simulink model "SistemaSeguimientoConIntegrador"  (R2020a)
settings: Solver=VariableStepAuto  StartTime=0.0  StopTime=10  RelTol=1e-3
settings Model: Creator=Sergio  LastModifiedBy=Sergio

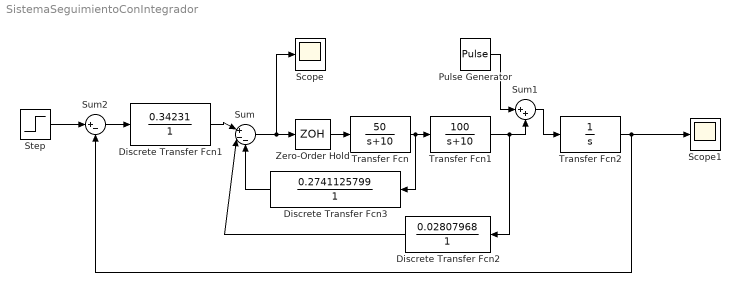
== system SistemaSeguimientoConIntegrador ==
  Discrete Transfer Fcn1 : DiscreteTransferFcn  Numerator=[0.34231]  Denominator=[1]
  Discrete Transfer Fcn2 : DiscreteTransferFcn  Numerator=[0.02807968]  Denominator=[1]
  Discrete Transfer Fcn3 : DiscreteTransferFcn  Numerator=[0.2741125799]  Denominator=[1]
  Pulse Generator : DiscretePulseGenerator  PulseType=Time based  Amplitude=0.1  Period=10
  Scope : Scope
  Scope1 : Scope
  Step : Step  SampleTime=0
  Sum : Sum  Inputs=|+--
  Sum1 : Sum  Inputs=|++
  Sum2 : Sum  Inputs=|+-
  Transfer Fcn : TransferFcn  Numerator=[50]  Denominator=[1 10]
  Transfer Fcn1 : TransferFcn  Numerator=[100]  Denominator=[1 10]
  Transfer Fcn2 : TransferFcn  Denominator=[1 0]
  Zero-Order Hold : ZeroOrderHold  SampleTime=0.02
  wires:
  Zero-Order Hold/1 -> Transfer Fcn/1
  Transfer Fcn/1 -> Discrete Transfer Fcn3/1, Transfer Fcn1/1
  Sum/1 -> Scope/1, Zero-Order Hold/1
  Transfer Fcn2/1 -> Sum2/2, Scope1/1
  Transfer Fcn1/1 -> Discrete Transfer Fcn2/1, Sum1/2
  Sum1/1 -> Transfer Fcn2/1
  Discrete Transfer Fcn3/1 -> Sum/3
  Discrete Transfer Fcn2/1 -> Sum/2
  Pulse Generator/1 -> Sum1/1
  Sum2/1 -> Discrete Transfer Fcn1/1
  Step/1 -> Sum2/1
  Discrete Transfer Fcn1/1 -> Sum/1
